simulink model "Modelo_Red_Mitigación_final"  (R2019b)
settings: Solver=VariableStepAuto  StartTime=0.0  StopTime=2.5  RelTol=1e-3
InitFcn:
  | Ts=20e-6;
undefined symbols (not defined in the file): D1, Delta, Ion, Lithium
libraries: powerlib x371, powerlib_meascontrol x286, simulink x50, simulink_extras x20, electricdrivelib x16
(part 3 of 11)

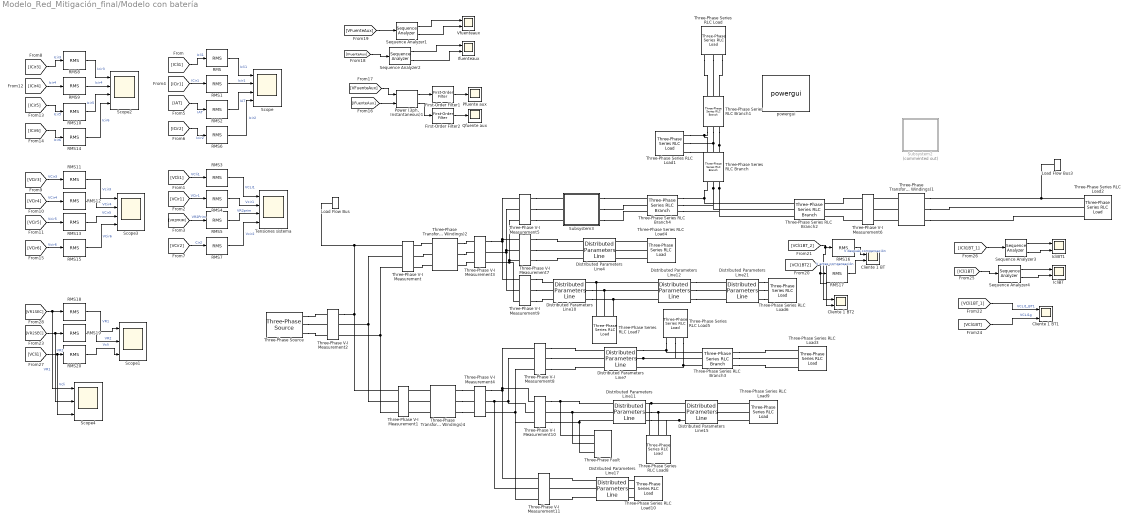
== system Modelo_Red_Mitigación_final/Modelo con batería  ==
  Cliente 1 BT : Scope  NumInputPorts=2
  Cliente 1 BT1 : Scope  NumInputPorts=3
  Cliente 1 BT2 : Scope  NumInputPorts=2
  Distributed Parameters Line10 : powerlib/Elements/Distributed Parameters Line  Phases=3  Frequency=60  Resistance=[0.213 0.639]  Inductance=[0.78e-3 2.35e-3]  Capacitance=[15e-9 15e-9]  Length=3  x1=[-2e-05 9.51822686756728e-10 32175.0070560474 -19325.063497857;-1e-05 9.56131340285843e-10 32247.6320174616 -19203.6295402535]  x2=[-2e-05 1.13231714803774e-09 31687.8811035516 -19346.7961292868;-1e-05 1.13823882988068e-09 31760.591456431 -19227.1984344754]  x3=[-2e-05 -7.26463476798207e-11 -137.471205101206 265.134927538951;-1e-05 -7.21901893651273e-11 -138.469760977224 264.614790455811]  x4=[-2e-05 7.73347694618198e-11 416.61303195894 -434.907199033177;-1e-05 7.69019064350013e-11 418.249629092397 -433.333518127755]  x5=1.78115131305569e-05  V1=ones(3,3)  V2=ones(3,3)  I1=ones(3,3)  I2=ones(3,3)  nHarmo=1  Measurements=None
      settings: SourceProductName=Simscape Electrical
  Distributed Parameters Line11 : powerlib/Elements/Distributed Parameters Line  Phases=3  Frequency=60  Resistance=[0.269 0.807]  Inductance=[0.85e-3 2.56e-3]  Capacitance=[15e-9 15e-9]  Length=18  x1=[-0.00012 -6.37664577338135e-10 31483.0427639002 -20454.4474545777;-0.00011 -6.37629545062547e-10 31559.9303096112 -20335.6141091962;-0.0001 -6.37585450659726e-10 31636.3693188544 -20216.4917497253;-9e-05 -6.37532294756353e-10 31712.3587052623 -20097.0820691573;-8e-05 -6.37470078107891e-10 31787.8973888575 -19977.3867645681;-7e-05 -6.37398801598575e-10 31862.9842960682 -19857.4075370929;-6e-05 -6.37318466241403e-10 31937.6183597431 -19737.1460919021;-5e-05 -6.37229073178117e-10 32011.7985191671 -19616.6041381771;-4e-05 -6.37130623679192e-10 32085.5237200758 -19495.7833890858;-3e-05 -6.37023119143813e-10 32158.792914671 -19374.6855617586;-2e-05 -6.36906561099856e-10 32231.6050616352 -19253.3123772635;-1e-05 -6.3678095120387e-10 32303.9591261466 -19131.6655605823]  x2=[-0.00012 -5.84352835995597e-10 29675.6367944872 -20128.6580942028;-0.00011 -5.8405713800106e-10 29751.3089897738 -20016.6408077542;-0.0001 -5.83753139261779e-10 29826.5583531049 -19904.3390405328;-9e-05 -5.83440844098248e-10 29901.3838150206 -19791.7543885953;-8e-05 -5.83120256948873e-10 29975.7843120855 -19678.8884520187;-7e-05 -5.82791382369907e-10 30049.7587869036 -19565.7428348779;-6e-05 -5.82454225035385e-10 30123.3061881342 -19452.3191452226;-5e-05 -5.8210878973706e-10 30196.4254705057 -19338.6189950544;-4e-05 -5.81755081384333e-10 30269.1155948313 -19224.6440003042;-3e-05 -5.81393105004181e-10 30341.3755280234 -19110.3957808088;-2e-05 -5.8102286574109e-10 30413.2042431086 -18995.8759602885;-1e-05 -5.80644368856979e-10 30484.6007192416 -18881.0861663232]  x3=[-0.00012 -2.40772351591986e-12 9.28421720698583 123.31084899492;-0.00011 -2.39518510900215e-12 8.81928138471592 123.344973326243;-0.0001 -2.38261266120228e-12 8.354220220936 123.37734465247;-9e-05 -2.37000635120258e-12 7.88904032519463 123.407962513534;-8e-05 -2.3573663581666e-12 7.42374830872781 123.436826474286;-7e-05 -2.34469286173662e-12 6.95835078436502 123.463936124505;-6e-05 -2.3319860420311e-12 6.49285436643523 123.489291078905;-5e-05 -2.31924607964205e-12 6.02726567067293 123.512890977134;-4e-05 -2.30647315563255e-12 5.56159131412406 123.534735483786;-3e-05 -2.29366745153411e-12 5.09583791505201 123.554824288401;-2e-05 -2.28082914934415e-12 4.63001209284352 123.573157105475;-1e-05 -2.26795843152334e-12 4.16412046791464 123.589733674456]  x4=[-0.00012 -5.10418440144233e-13 241.702417431104 -294.296225052447;-0.00011 -5.2378075498003e-13 242.810167870242 -293.382939263662;-0.0001 -5.37135625731908e-13 243.914467439433 -292.465483853906;-9e-05 -5.50482862597592e-13 245.015300444135 -291.54387186225;-8e-05 -5.63822275883302e-13 246.112651239076 -290.618116386841;-7e-05 -5.77153676006447e-13 247.206504228471 -289.688230584714;-6e-05 -5.90476873498324e-13 248.296843866248 -288.754227671603;-5e-05 -6.03791679006805e-13 249.383654656268 -287.816120921758;-4e-05 -6.17097903299031e-13 250.466921152542 -286.873923667753;-3e-05 -6.30395357264102e-13 251.546627959458 -285.927649300295;-2e-05 -6.43683851915763e-13 252.62275973199 -284.977311268038;-1e-05 -6.5696319839509e-13 253.695301175924 -284.02292307739]  x5=0.000111541920370774  V1=ones(3,3)  V2=ones(3,3)  I1=ones(3,3)  I2=ones(3,3)  nHarmo=1  Measurements=None
      settings: SourceProductName=Simscape Electrical
  Distributed Parameters Line12 : powerlib/Elements/Distributed Parameters Line  Phases=3  Frequency=60  Resistance=[0.269 0.807]  Inductance=[0.85e-3 2.56e-3]  Capacitance=[15e-9 15e-9]  Length=6  x1=[-4e-05 1.12225551603288e-09 0 0;-3e-05 1.12820660384581e-09 31614.7203957403 -19466.1188633009;-2e-05 1.1341416573456e-09 31687.8811035516 -19346.7961292868;-1e-05 1.14006059218202e-09 31760.591456431 -19227.1984344754]  x2=[-4e-05 8.82977482669238e-10 0 0;-3e-05 8.896258470369e-10 30837.5027565975 -19380.3404703214;-2e-05 8.96261567852084e-10 30910.3456112432 -19263.9483803878;-1e-05 9.0288455080651e-10 30982.7491614575 -19147.2825071068]  x3=[-4e-05 -3.70011263341918e-11 0 0;-3e-05 -3.70159507502131e-11 -40.5019848242572 176.337783353315;-2e-05 -3.70302490876394e-11 -41.1664732198487 176.183841754301;-1e-05 -3.70440211432594e-11 -41.8303765487335 176.027396192912]  x4=[-4e-05 3.94498278114461e-11 0 0;-3e-05 3.94988779511581e-11 300.866672819828 -339.753955836193;-2e-05 3.95473667243833e-11 302.145374033219 -338.617303560145;-1e-05 3.95952934419892e-11 303.419781092044 -337.475838782682]  x5=3.71806401235912e-05  V1=ones(3,3)  V2=ones(3,3)  I1=ones(3,3)  I2=ones(3,3)  nHarmo=1  Measurements=None
      settings: SourceProductName=Simscape Electrical
  Distributed Parameters Line15 : powerlib/Elements/Distributed Parameters Line  Phases=3  Frequency=60  Resistance=[0.269 0.807]  Inductance=[0.85e-3 2.56e-3]  Capacitance=[15e-9 15e-9]  Length=12  x1=[-8e-05 -5.81290096062597e-10 0 0;-7e-05 -5.80962527082388e-10 0 0;-6e-05 -5.80626701338705e-10 0 0;-5e-05 -5.80282623604376e-10 30196.4254705057 -19338.6189950544;-4e-05 -5.79930298769507e-10 30269.1155948313 -19224.6440003042;-3e-05 -5.79569731841414e-10 30341.3755280234 -19110.3957808088;-2e-05 -5.7920092794455e-10 30413.2042431086 -18995.8759602885;-1e-05 -5.78823892320436e-10 30484.6007192416 -18881.0861663232]  x2=[-8e-05 -5.1837948200219e-10 0 0;-7e-05 -5.17954517458826e-10 0 0;-6e-05 -5.17522191635274e-10 0 0;-5e-05 -5.17082510675841e-10 29816.1536069767 -19273.9878791668;-4e-05 -5.16635480829367e-10 29888.6027805653 -19161.4469314478;-3e-05 -5.16181108449134e-10 29960.6271709498 -19048.633657154;-2e-05 -5.15719399992781e-10 30032.2257545041 -18935.5496596116;-1e-05 -5.15250362022206e-10 30103.3975136541 -18822.1965459946]  x3=[-8e-05 6.30193856587518e-13 0 0;-7e-05 6.47027122188518e-13 0 0;-6e-05 6.63851192101914e-13 0 0;-5e-05 6.80665827220432e-13 86.3403246372238 -15.5892894445521;-4e-05 6.97470788570887e-13 86.3984811910831 -15.2636840808927;-3e-05 7.14265837317582e-13 86.4554098312811 -14.9378617864961;-2e-05 7.31050734765698e-13 86.511109748736 -14.6118271920186;-1e-05 7.47825242364687e-13 86.5655801518285 -14.2855849311333]  x4=[-8e-05 -2.76869898482782e-12 0 0;-7e-05 -2.78266132861739e-12 0 0;-6e-05 -2.79658412463005e-12 0 0;-5e-05 -2.81046717499204e-12 161.912076262647 -146.998141908733;-4e-05 -2.82431028239449e-12 162.465094324739 -146.38670462291;-3e-05 -2.8381132500962e-12 163.015803398223 -145.773186857987;-2e-05 -2.85187588192645e-12 163.564195656305 -145.157597333408;-1e-05 -2.86559798228777e-12 164.110263305116 -144.539944798065]  x5=7.43612802471824e-05  V1=ones(3,3)  V2=ones(3,3)  I1=ones(3,3)  I2=ones(3,3)  nHarmo=1  Measurements=None
      settings: SourceProductName=Simscape Electrical
  Distributed Parameters Line17 : powerlib/Elements/Distributed Parameters Line  Phases=3  Frequency=60  Resistance=[0.213 0.639]  Inductance=[0.78e-3 2.35e-3]  Capacitance=[15e-9 15e-9]  Length=18  x1=[-0.00011 -6.37629545062547e-10 31559.9303096112 -20335.6141091962;-0.0001 -6.37585450659726e-10 31636.3693188544 -20216.4917497253;-9e-05 -6.37532294756353e-10 31712.3587052623 -20097.0820691573;-8e-05 -6.37470078107891e-10 31787.8973888575 -19977.3867645681;-7e-05 -6.37398801598575e-10 31862.9842960682 -19857.4075370929;-6e-05 -6.37318466241403e-10 31937.6183597431 -19737.1460919021;-5e-05 -6.37229073178117e-10 32011.7985191671 -19616.6041381771;-4e-05 -6.37130623679192e-10 32085.5237200758 -19495.7833890858;-3e-05 -6.37023119143813e-10 32158.792914671 -19374.6855617586;-2e-05 -6.36906561099856e-10 32231.6050616352 -19253.3123772635;-1e-05 -6.3678095120387e-10 32303.9591261466 -19131.6655605823]  x2=[-0.00011 -5.81093394391643e-10 30839.7793585654 -20381.2716559516;-0.0001 -5.80562463791867e-10 30916.3956097666 -20264.8638707272;-9e-05 -5.80023282114402e-10 30992.5724705526 -20148.1680769308;-8e-05 -5.79475857022214e-10 31068.3088582815 -20031.1859330679;-7e-05 -5.78920196295424e-10 31143.6036965717 -19913.9191017138;-6e-05 -5.78356307831202e-10 31218.4559153168 -19796.3692494898;-5e-05 -5.77784199643652e-10 31292.8644507012 -19678.5380470393;-4e-05 -5.77203879863696e-10 31366.8282452148 -19560.4271690046;-3e-05 -5.76615356738963e-10 31440.3462476684 -19442.0382940027;-2e-05 -5.7601863863367e-10 31513.4174132084 -19323.3731046016;-1e-05 -5.75413734028501e-10 31586.0407033319 -19204.4332872963]  x3=[-0.00011 -5.33423696024894e-12 65.9317893508074 -5.21472769212498;-0.0001 -5.30896708029375e-12 65.9509798461571 -4.96613423439622;-9e-05 -5.28362174816493e-12 65.9692330321003 -4.71747019690742;-8e-05 -5.25820132407573e-12 65.9865486492189 -4.46873911372498;-7e-05 -5.23270616930667e-12 66.0029264514196 -4.21994451986815;-6e-05 -5.20713664620032e-12 66.0183662059376 -3.97108995125883;-5e-05 -5.1814931181562e-12 66.0328676933398 -3.72217894467127;-4e-05 -5.15577594962561e-12 66.046430707528 -3.47321503768184;-3e-05 -5.12998550610644e-12 66.0590550557418 -3.22420176861875;-2e-05 -5.10412215413798e-12 66.0707405585611 -2.97514267651174;-1e-05 -5.0781862612957e-12 66.0814870499091 -2.72604130104181]  x4=[-0.00011 2.08995199063691e-12 202.227351702482 -174.253957712764;-0.0001 2.06944266433478e-12 202.882835041371 -173.490342096433;-9e-05 2.04890392667166e-12 203.535434966092 -172.724260798319;-8e-05 2.02833606954849e-12 204.185142201756 -171.955724706133;-7e-05 2.00773938528004e-12 204.831947514583 -171.184744742474;-6e-05 1.98711416659078e-12 205.47584171204 -170.411331864673;-5e-05 1.96646070661072e-12 206.116815642964 -169.635497064641;-4e-05 1.94577929887126e-12 206.754860197698 -168.857251368706;-3e-05 1.92507023730096e-12 207.389966308214 -168.076605837463;-2e-05 1.90433381622144e-12 208.022124948251 -167.293571565612;-1e-05 1.88357033034313e-12 208.651327133435 -166.508159681805]  x5=0.000106869078783341  V1=ones(3,3)  V2=ones(3,3)  I1=ones(3,3)  I2=ones(3,3)  nHarmo=1  Measurements=None
      settings: SourceProductName=Simscape Electrical
  Distributed Parameters Line21 : powerlib/Elements/Distributed Parameters Line  Phases=3  Frequency=60  Resistance=[0.269 0.807]  Inductance=[0.85e-3 2.56e-3]  Capacitance=[15e-9 15e-9]  Length=3  x1=[-2e-05 8.96265853704287e-10 30910.3456112432 -19263.9483803878;-1e-05 9.02886693747839e-10 30982.7491614575 -19147.2825071068]  x2=[-2e-05 8.82848388597059e-10 30521.2143172031 -19221.4149453175;-1e-05 8.88901904202634e-10 30593.4602857332 -19106.2163612263]  x3=[-2e-05 3.05576494227813e-11 -43.7280619985849 177.821448028189;-1e-05 3.04685047093702e-11 -44.3981207401299 177.655333890483]  x4=[-2e-05 -2.43827173429009e-11 300.811121285802 -339.602032284589;-1e-05 -2.42495845607924e-11 302.089250157008 -338.465590511979]  x5=1.85903200617956e-05  V1=ones(3,3)  V2=ones(3,3)  I1=ones(3,3)  I2=ones(3,3)  nHarmo=1  Measurements=None
      settings: SourceProductName=Simscape Electrical
  Distributed Parameters Line4 : powerlib/Elements/Distributed Parameters Line  Phases=3  Frequency=60  Resistance=[0.213 0.639]  Inductance=[0.78e-3 2.35e-3]  Capacitance=[15e-9 15e-9]  Length=9  x1=[-6e-05 9.27062321547884e-10 31879.9448487023 -19808.0356092313;-5e-05 9.31443643683125e-10 31954.3926645116 -19687.7105752571;-4e-05 9.35811727942434e-10 32028.3863376699 -19567.1057353368;-3e-05 9.40166512245665e-10 32101.9248165634 -19446.2228035321;-2e-05 9.44507934701694e-10 32175.0070560474 -19325.063497857;-1e-05 9.48835933609296e-10 32247.6320174616 -19203.6295402535]  x2=[-6e-05 9.30715846640024e-10 31220.754132217 -19854.1863402283;-5e-05 9.36913847546258e-10 31295.3806160507 -19736.3460628703;-4e-05 9.43098532832856e-10 31369.5623232534 -19618.2252883483;-3e-05 9.49269814601747e-10 31443.2981995388 -19499.8256954198;-2e-05 9.5542760514536e-10 31516.5871969568 -19381.1489668053;-1e-05 9.61571816947859e-10 31589.4282739087 -19262.1967891637]  x3=[-6e-05 -3.66911385239073e-11 9.19435123998005 67.3100361697751;-5e-05 -3.65713742858999e-11 8.94053364683108 67.3442196629408;-4e-05 -3.64510902877129e-11 8.68658898890908 67.3774460456783;-3e-05 -3.63302882388482e-11 8.43252087532973 67.4097148457672;-2e-05 -3.62089698561704e-11 8.17833291696331 67.4410256045963;-1e-05 -3.60871368638822e-11 7.92402872638336 67.4713778771705]  x4=[-6e-05 4.05346197813055e-11 264.776860672235 -241.746580654789;-5e-05 4.04416044214767e-11 265.686340119028 -240.74667989379;-4e-05 4.03480142969314e-11 266.59204357483 -239.743357589577;-3e-05 4.02538507377923e-11 267.49395816759 -238.736628001579;-2e-05 4.01591150823322e-11 268.392071079105 -237.726505437652;-1e-05 4.00638086769543e-11 269.286369545202 -236.713004253875]  x5=5.34345393916706e-05  V1=ones(3,3)  V2=ones(3,3)  I1=ones(3,3)  I2=ones(3,3)  nHarmo=1  Measurements=None
      settings: SourceProductName=Simscape Electrical
  Distributed Parameters Line7 : powerlib/Elements/Distributed Parameters Line  Phases=3  Frequency=60  Resistance=[0.213 0.639]  Inductance=[0.78e-3 2.35e-3]  Capacitance=[15e-9 15e-9]  Length=4.4  x1=[-3e-05 -6.37023119143813e-10 0 0;-2e-05 -6.36906561099856e-10 32231.6050616352 -19253.3123772635;-1e-05 -6.3678095120387e-10 32303.9591261466 -19131.6655605823]  x2=[-3e-05 -6.20206594908238e-10 0 0;-2e-05 -6.19631999252479e-10 31928.0322823366 -19306.2030459998;-1e-05 -6.19048597254452e-10 32000.58789672 -19185.700293177]  x3=[-3e-05 -2.2707610684769e-11 0 0;-2e-05 -2.26378782855031e-11 2.67417656215666 49.6193899931641;-1e-05 -2.25678241518777e-11 2.48709730897001 49.6291187767325]  x4=[-3e-05 1.89896750235836e-11 0 0;-2e-05 1.89284208409242e-11 277.339936666534 -218.99027498491;-1e-05 1.88668976435065e-11 278.163537790718 -217.943174364135]  x5=2.61235525914834e-05  V1=ones(3,3)  V2=ones(3,3)  I1=ones(3,3)  I2=ones(3,3)  nHarmo=1  Measurements=None
      settings: SourceProductName=Simscape Electrical
  First-Order Filter1 : powerlib_meascontrol/Filters/First-Order Filter  FilterType=Lowpass  Tc=10e-3  Ts=0  Initialize=on  Vac_Init=[0, 0, 60]  Vdc_Init=0  PlotResponse=off  FreqRange="[0,  200,  1]"
      settings: SourceProductName=Simscape Electrical
  First-Order Filter2 : powerlib_meascontrol/Filters/First-Order Filter  FilterType=Lowpass  Tc=10e-3  Ts=0  Initialize=on  Vac_Init=[0, 0, 60]  Vdc_Init=0  PlotResponse=off  FreqRange="[0,  200,  1]"
      settings: SourceProductName=Simscape Electrical
  IcliBT : Scope  NumInputPorts=2
  IcliBT1 : Scope  NumInputPorts=2
  Ifuenteaux : Scope  NumInputPorts=2
  Load Flow Bus : powerlib/Measurements/Load Flow Bus  LConnTagsString=a  Phases=single  Connectors=on one side  ID=BUS_1  Vbase=115e3  Vref=1.05  Vangle=0  VLF=1  VLFb=1  VLFc=1  angleLF=0  angleLFb=0  angleLFc=0
      settings: SourceProductName=Simscape Electrical
  Load Flow Bus3 : powerlib/Measurements/Load Flow Bus  LConnTagsString=a  Phases=single  Connectors=on one side  ID=BUS_4  Vbase=440  Vref=1  Vangle=0  VLF=0.9785  VLFb=1  VLFc=1  angleLF=28.33  angleLFb=0  angleLFc=0
      settings: SourceProductName=Simscape Electrical
  "Pfuente aux " : Scope
  "Power (3ph, Instantaneous)1" : powerlib_meascontrol/Measurements/Power (3ph, Instantaneous)
      settings: SourceProductName=Simscape Electrical
  Qfuente aux : Scope
  RMS{,1..20} (21 alike) : powerlib_meascontrol/Measurements/RMS  TrueRMS=on  Freq=60  RMSInit=120  Ts=0
      settings: SourceProductName=Simscape Electrical
  Scope : Scope  NumInputPorts=4
  Scope1 : Scope  NumInputPorts=3
  Scope2 : Scope  NumInputPorts=4
  Scope3 : Scope  NumInputPorts=4
  Scope4 : Scope  NumInputPorts=3
  Sequence Analyzer{1..4} (4 alike) : powerlib_meascontrol/Measurements/Sequence Analyzer  Freq=60  n=1  seq=Positive Negative Zero  InInit=[1, 0]  Ts=0
      settings: SourceProductName=Simscape Electrical  SourceProductBaseCode=PS
  Subsystem2 : Subsystem  Commented=on
  Subsystem3 : Subsystem
  Tensiones sistema : Scope  NumInputPorts=4
  Three-Phase Series RLC Branch : powerlib/Elements/Three-Phase Series RLC Branch  LConnTagsString=A|B|C  RConnTagsString=A|B|C  BranchType=RL  Resistance=0.213  Inductance=0.78e-3  Capacitance=1e-6  Measurements=None
      settings: SourceProductName=Simscape Electrical
  Three-Phase Series RLC Branch1 : powerlib/Elements/Three-Phase Series RLC Branch  LConnTagsString=A|B|C  RConnTagsString=A|B|C  BranchType=RL  Resistance=0.213  Inductance=0.78e-3  Capacitance=1e-6  Measurements=None
      settings: SourceProductName=Simscape Electrical
  Three-Phase Series RLC Branch2 : powerlib/Elements/Three-Phase Series RLC Branch  LConnTagsString=A|B|C  RConnTagsString=A|B|C  BranchType=RL  Resistance=0.213*1.7  Inductance=0.78e-3*1.7  Capacitance=1e-6  Measurements=None
      settings: SourceProductName=Simscape Electrical
  Three-Phase Series RLC Branch3 : powerlib/Elements/Three-Phase Series RLC Branch  LConnTagsString=A|B|C  RConnTagsString=A|B|C  BranchType=RL  Resistance=0.213*2.2  Inductance=0.78e-3*2.2  Capacitance=1e-6  Measurements=None
      settings: SourceProductName=Simscape Electrical
  Three-Phase Series RLC Branch4 : powerlib/Elements/Three-Phase Series RLC Branch  LConnTagsString=A|B|C  RConnTagsString=A|B|C  BranchType=RL  Resistance=0.213*7  Inductance=0.78e-3*7  Capacitance=1e-6  Measurements=None
      settings: SourceProductName=Simscape Electrical
  Three-Phase Series RLC Load : powerlib/Elements/Three-Phase Series RLC Load  LConnTagsString=A|B|C  Configuration=Y (grounded)  NominalVoltage=34.5e3  Vabc=[1e3 1e3 1e3]  Vabcp=[1e3 1e3 1e3]  NominalFrequency=60  UnbalancedPower=off  ActivePower=0.5e6  InductivePower=0.1e6  CapacitivePower=0  Pabc=[10e3 9e3 11e3]  QLabc=[100 90 110]  QCabc=[100 90 110]  Pabcp=[10e3 9e3 11e3]  QLabcp=[100 90 110]  QCabcp=[100 90 110]  Measurements=None  LoadType=constant Z
      settings: SourceProductName=Simscape Electrical
  Three-Phase Series RLC Load1 : powerlib/Elements/Three-Phase Series RLC Load  LConnTagsString=A|B|C  Configuration=Y (grounded)  NominalVoltage=34.5e3  Vabc=[1e3 1e3 1e3]  Vabcp=[1e3 1e3 1e3]  NominalFrequency=60  UnbalancedPower=off  ActivePower=2.5e6  InductivePower=1e6  CapacitivePower=0  Pabc=[10e3 9e3 11e3]  QLabc=[100 90 110]  QCabc=[100 90 110]  Pabcp=[10e3 9e3 11e3]  QLabcp=[100 90 110]  QCabcp=[100 90 110]  Measurements=None  LoadType=constant Z
      settings: SourceProductName=Simscape Electrical
  Three-Phase Series RLC Load10 : powerlib/Elements/Three-Phase Series RLC Load  LConnTagsString=A|B|C  Configuration=Y (grounded)  NominalVoltage=34.5e3  Vabc=[1e3 1e3 1e3]  Vabcp=[1e3 1e3 1e3]  NominalFrequency=60  UnbalancedPower=off  ActivePower=3.4e6  InductivePower=1.1e6  CapacitivePower=0  Pabc=[10e3 9e3 11e3]  QLabc=[100 90 110]  QCabc=[100 90 110]  Pabcp=[10e3 9e3 11e3]  QLabcp=[100 90 110]  QCabcp=[100 90 110]  Measurements=None  LoadType=constant Z
      settings: SourceProductName=Simscape Electrical
  Three-Phase Series RLC Load2 : powerlib/Elements/Three-Phase Series RLC Load  LConnTagsString=A|B|C  Configuration=Y (grounded)  NominalVoltage=440  Vabc=[1e3 1e3 1e3]  Vabcp=[1e3 1e3 1e3]  NominalFrequency=60  UnbalancedPower=off  ActivePower=6.5e6  InductivePower=3e6  CapacitivePower=0  Pabc=[10e3 9e3 11e3]  QLabc=[100 90 110]  QCabc=[100 90 110]  Pabcp=[10e3 9e3 11e3]  QLabcp=[100 90 110]  QCabcp=[100 90 110]  Measurements=None  LoadType=constant Z
      settings: SourceProductName=Simscape Electrical
  Three-Phase Series RLC Load3 : powerlib/Elements/Three-Phase Series RLC Load  LConnTagsString=A|B|C  Configuration=Y (grounded)  NominalVoltage=34.5e3  Vabc=[1e3 1e3 1e3]  Vabcp=[1e3 1e3 1e3]  NominalFrequency=60  UnbalancedPower=off  ActivePower=3e6  InductivePower=0.7e6  CapacitivePower=0  Pabc=[10e3 9e3 11e3]  QLabc=[100 90 110]  QCabc=[100 90 110]  Pabcp=[10e3 9e3 11e3]  QLabcp=[100 90 110]  QCabcp=[100 90 110]  Measurements=None  LoadType=constant Z
      settings: SourceProductName=Simscape Electrical
  Three-Phase Series RLC Load4 : powerlib/Elements/Three-Phase Series RLC Load  LConnTagsString=A|B|C  Configuration=Y (grounded)  NominalVoltage=34.5e3  Vabc=[1e3 1e3 1e3]  Vabcp=[1e3 1e3 1e3]  NominalFrequency=60  UnbalancedPower=off  ActivePower=6.2e6  InductivePower=2e6  CapacitivePower=0  Pabc=[10e3 9e3 11e3]  QLabc=[100 90 110]  QCabc=[100 90 110]  Pabcp=[10e3 9e3 11e3]  QLabcp=[100 90 110]  QCabcp=[100 90 110]  Measurements=None  LoadType=constant Z
      settings: SourceProductName=Simscape Electrical
  Three-Phase Series RLC Load5 : powerlib/Elements/Three-Phase Series RLC Load  LConnTagsString=A|B|C  Configuration=Y (grounded)  NominalVoltage=34.5e3  Vabc=[1e3 1e3 1e3]  Vabcp=[1e3 1e3 1e3]  NominalFrequency=60  UnbalancedPower=off  ActivePower=3e6  InductivePower=0.7e6  CapacitivePower=0  Pabc=[10e3 9e3 11e3]  QLabc=[100 90 110]  QCabc=[100 90 110]  Pabcp=[10e3 9e3 11e3]  QLabcp=[100 90 110]  QCabcp=[100 90 110]  Measurements=None  LoadType=constant Z
      settings: SourceProductName=Simscape Electrical
  Three-Phase Series RLC Load6 : powerlib/Elements/Three-Phase Series RLC Load  LConnTagsString=A|B|C  Configuration=Y (grounded)  NominalVoltage=34.5e3  Vabc=[1e3 1e3 1e3]  Vabcp=[1e3 1e3 1e3]  NominalFrequency=60  UnbalancedPower=off  ActivePower=9.4e6  InductivePower=4.2e6  CapacitivePower=0  Pabc=[10e3 9e3 11e3]  QLabc=[100 90 110]  QCabc=[100 90 110]  Pabcp=[10e3 9e3 11e3]  QLabcp=[100 90 110]  QCabcp=[100 90 110]  Measurements=None  LoadType=constant Z
      settings: SourceProductName=Simscape Electrical
  Three-Phase Series RLC Load7 : powerlib/Elements/Three-Phase Series RLC Load  LConnTagsString=A|B|C  Configuration=Y (grounded)  NominalVoltage=34.5e3  Vabc=[1e3 1e3 1e3]  Vabcp=[1e3 1e3 1e3]  NominalFrequency=60  UnbalancedPower=off  ActivePower=4.4e6  InductivePower=0.8e6  CapacitivePower=0  Pabc=[10e3 9e3 11e3]  QLabc=[100 90 110]  QCabc=[100 90 110]  Pabcp=[10e3 9e3 11e3]  QLabcp=[100 90 110]  QCabcp=[100 90 110]  Measurements=None  LoadType=constant Z
      settings: SourceProductName=Simscape Electrical
  Three-Phase Series RLC Load8 : powerlib/Elements/Three-Phase Series RLC Load  LConnTagsString=A|B|C  Configuration=Y (grounded)  NominalVoltage=34.5e3  Vabc=[1e3 1e3 1e3]  Vabcp=[1e3 1e3 1e3]  NominalFrequency=60  UnbalancedPower=off  ActivePower=5e6  InductivePower=2.5e6  CapacitivePower=0  Pabc=[10e3 9e3 11e3]  QLabc=[100 90 110]  QCabc=[100 90 110]  Pabcp=[10e3 9e3 11e3]  QLabcp=[100 90 110]  QCabcp=[100 90 110]  Measurements=None  LoadType=constant Z
      settings: SourceProductName=Simscape Electrical
  Three-Phase Series RLC Load9 : powerlib/Elements/Three-Phase Series RLC Load  LConnTagsString=A|B|C  Configuration=Y (grounded)  NominalVoltage=34.5e3  Vabc=[1e3 1e3 1e3]  Vabcp=[1e3 1e3 1e3]  NominalFrequency=60  UnbalancedPower=off  ActivePower=2.3e6  InductivePower=1.2e6  CapacitivePower=0  Pabc=[10e3 9e3 11e3]  QLabc=[100 90 110]  QCabc=[100 90 110]  Pabcp=[10e3 9e3 11e3]  QLabcp=[100 90 110]  QCabcp=[100 90 110]  Measurements=None  LoadType=constant Z
      settings: SourceProductName=Simscape Electrical
  Three-Phase V-I Measurement : powerlib/Measurements/Three-Phase V-I Measurement  VoltageMeasurement=phase-to-ground  SetLabelV=on  LabelV=VR2PRIM  Vpu=off  VpuLL=off  CurrentMeasurement=yes  SetLabelI=on  LabelI=IR2PRIM  Ipu=off  Pbase=100e6  Vbase=500e3  OutputType=Complex  PhasorSimulation=off  PSBequivalent=0
      settings: SourceProductName=Simscape Electrical
  Three-Phase V-I Measurement1 : powerlib/Measurements/Three-Phase V-I Measurement  VoltageMeasurement=phase-to-ground  SetLabelV=on  LabelV=VR1PRIM  Vpu=off  VpuLL=off  CurrentMeasurement=yes  SetLabelI=on  LabelI=IR1PRIM  Ipu=off  Pbase=100e6  Vbase=500e3  OutputType=Complex  PhasorSimulation=off  PSBequivalent=0
      settings: SourceProductName=Simscape Electrical
  Three-Phase V-I Measurement10 : powerlib/Measurements/Three-Phase V-I Measurement  VoltageMeasurement=phase-to-ground  SetLabelV=on  LabelV=VCir5  Vpu=off  VpuLL=off  CurrentMeasurement=yes  SetLabelI=on  LabelI=ICir5  Ipu=off  Pbase=100e6  Vbase=500e3  OutputType=Complex  PhasorSimulation=off  PSBequivalent=0
      settings: SourceProductName=Simscape Electrical
  Three-Phase V-I Measurement11 : powerlib/Measurements/Three-Phase V-I Measurement  VoltageMeasurement=phase-to-ground  SetLabelV=on  LabelV=VCir6  Vpu=off  VpuLL=off  CurrentMeasurement=yes  SetLabelI=on  LabelI=ICir6  Ipu=off  Pbase=100e6  Vbase=500e3  OutputType=Complex  PhasorSimulation=off  PSBequivalent=0
      settings: SourceProductName=Simscape Electrical
  Three-Phase V-I Measurement2 : powerlib/Measurements/Three-Phase V-I Measurement  VoltageMeasurement=phase-to-ground  SetLabelV=on  LabelV=VAT  Vpu=off  VpuLL=off  CurrentMeasurement=yes  SetLabelI=on  LabelI=IAT  Ipu=off  Pbase=100e6  Vbase=500e3  OutputType=Complex  PhasorSimulation=off  PSBequivalent=0
      settings: SourceProductName=Simscape Electrical
  Three-Phase V-I Measurement3 : powerlib/Measurements/Three-Phase V-I Measurement  VoltageMeasurement=phase-to-ground  SetLabelV=on  LabelV=VR2SEC  Vpu=off  VpuLL=off  CurrentMeasurement=yes  SetLabelI=on  LabelI=IR2SEC  Ipu=off  Pbase=100e6  Vbase=500e3  OutputType=Complex  PhasorSimulation=off  PSBequivalent=0
      settings: SourceProductName=Simscape Electrical
  Three-Phase V-I Measurement4 : powerlib/Measurements/Three-Phase V-I Measurement  VoltageMeasurement=phase-to-ground  SetLabelV=on  LabelV=VR1SEC  Vpu=off  VpuLL=off  CurrentMeasurement=yes  SetLabelI=on  LabelI=IR1SEC  Ipu=off  Pbase=100e6  Vbase=500e3  OutputType=Complex  PhasorSimulation=off  PSBequivalent=0
      settings: SourceProductName=Simscape Electrical
  Three-Phase V-I Measurement5 : powerlib/Measurements/Three-Phase V-I Measurement  VoltageMeasurement=phase-to-ground  SetLabelV=on  LabelV=VCir1  Vpu=off  VpuLL=off  CurrentMeasurement=yes  SetLabelI=on  LabelI=ICir1  Ipu=off  Pbase=100e6  Vbase=500e3  OutputType=Complex  PhasorSimulation=off  PSBequivalent=0
      settings: SourceProductName=Simscape Electrical
  Three-Phase V-I Measurement6 : powerlib/Measurements/Three-Phase V-I Measurement  VoltageMeasurement=phase-to-ground  SetLabelV=on  LabelV=VCli1  Vpu=off  VpuLL=off  CurrentMeasurement=yes  SetLabelI=on  LabelI=ICli1  Ipu=off  Pbase=100e6  Vbase=500e3  OutputType=Complex  PhasorSimulation=off  PSBequivalent=0
      settings: SourceProductName=Simscape Electrical
  Three-Phase V-I Measurement7 : powerlib/Measurements/Three-Phase V-I Measurement  VoltageMeasurement=phase-to-ground  SetLabelV=on  LabelV=VCir2  Vpu=off  VpuLL=off  CurrentMeasurement=yes  SetLabelI=on  LabelI=ICir2  Ipu=off  Pbase=100e6  Vbase=500e3  OutputType=Complex  PhasorSimulation=off  PSBequivalent=0
      settings: SourceProductName=Simscape Electrical
  Three-Phase V-I Measurement8 : powerlib/Measurements/Three-Phase V-I Measurement  VoltageMeasurement=phase-to-ground  SetLabelV=on  LabelV=VCir4  Vpu=off  VpuLL=off  CurrentMeasurement=yes  SetLabelI=on  LabelI=ICir4  Ipu=off  Pbase=100e6  Vbase=500e3  OutputType=Complex  PhasorSimulation=off  PSBequivalent=0
      settings: SourceProductName=Simscape Electrical
  Three-Phase V-I Measurement9 : powerlib/Measurements/Three-Phase V-I Measurement  VoltageMeasurement=phase-to-ground  SetLabelV=on  LabelV=VCir3  Vpu=off  VpuLL=off  CurrentMeasurement=yes  SetLabelI=on  LabelI=ICir3  Ipu=off  Pbase=100e6  Vbase=500e3  OutputType=Complex  PhasorSimulation=off  PSBequivalent=0
      settings: SourceProductName=Simscape Electrical
  Three-Phase Fault : powerlib/Elements/Three-Phase Fault  InitialStates=0  FaultA=on  FaultB=on  FaultC=on  GroundFault=off  SwitchTimes=[0.2,0.4]  External=off  SwitchStatus=NaN  FaultResistance=0.3  GroundResistance=0.01  SnubberResistance=1e6  SnubberCapacitance=inf  Measurements=None
      settings: SourceProductName=Simscape Electrical
  Three-Phase Source : powerlib/Electrical Sources/Three-Phase Source  InternalConnection=Yg  VoltagePhases=off  Voltage=(115000)*1.39942  PhaseAngle=16.7311  Voltage_phases=[25e3 25e3 25e3]/sqrt(3)  PhaseAngles_phases=[0 -120 +120]  Frequency=60  NonIdealSource=on  SpecifyImpedance=on  Resistance=0.8929  Inductance=16.58e-3  ShortCircuitLevel=100e6  BaseVoltage=115e3  XRratio=5.946  BusType=swing  Pref=10e3  Qref=0  Prefabc=[10e3, 10e3, 10e3]  Qrefabc=[0, 0, 0]  Qmin=-inf  Qmax=inf
      settings: SourceProductName=Simscape Electrical
  Three-Phase Transformer Inductance Matrix Type (Two Windings)1 : powerlib/Elements/Three-Phase Transformer Inductance Matrix Type (Two Windings)  CoreType=Three-limb or five-limb core  Winding1Connection=Yg  Winding2Connection=Yg  AutoTransformer=off  Measurements=None  NominalPower=[10e6, 60]  VLLnom=[34.5e3, 440]  WindingResistances=[0.01, 0.01]  NoLoadIexcPos=2  NoLoadPlossPos=1000  ShortCircuitReactancePos=0.06  ShortCircuitReactancePosAuto=0.06  NoLoadIexcZero=100  NoLoadPlossZero=500000  ShortCircuitReactanceZero=0.03  ShortCircuitReactanceZeroAuto=0.03
      settings: SourceProductName=Simscape Electrical  SourceProductBaseCode=PS
  Three-Phase Transformer Inductance Matrix Type (Two Windings)2 : powerlib/Elements/Three-Phase Transformer Inductance Matrix Type (Two Windings)  CoreType=Three single-phase cores  Winding1Connection=Delta (D1)  Winding2Connection=Y  AutoTransformer=off  Measurements=None  NominalPower=[40e6, 60]  VLLnom=[115e3, 34.5e3]  WindingResistances=[0.006, 0.006]  NoLoadIexcPos=2  NoLoadPlossPos=16600  ShortCircuitReactancePos=0.1056  ShortCircuitReactancePosAuto=0.06  NoLoadIexcZero=100  NoLoadPlossZero=500000  ShortCircuitReactanceZero=0.1056  ShortCircuitReactanceZeroAuto=0.03
      settings: SourceProductName=Simscape Electrical  SourceProductBaseCode=PS
  Three-Phase Transformer Inductance Matrix Type (Two Windings)4 : powerlib/Elements/Three-Phase Transformer Inductance Matrix Type (Two Windings)  CoreType=Three single-phase cores  Winding1Connection=Delta (D1)  Winding2Connection=Y  AutoTransformer=off  Measurements=None  NominalPower=[30e6, 60]  VLLnom=[115e3, 34.5e3]  WindingResistances=[0.006, 0.006]  NoLoadIexcPos=2  NoLoadPlossPos=14300  ShortCircuitReactancePos=0.0912  ShortCircuitReactancePosAuto=0.06  NoLoadIexcZero=100  NoLoadPlossZero=500000  ShortCircuitReactanceZero=0.0912  ShortCircuitReactanceZeroAuto=0.03
      settings: SourceProductName=Simscape Electrical  SourceProductBaseCode=PS
  Vfuenteaux : Scope  NumInputPorts=2
  powergui : powerlib/powergui  Priority=1  SimulationMode=Discrete  SampleTime=10e-6  frequency=60  Iterations=50  frequencyindice=0  Pbase=100e6  ErrMax=0.0001  UnitsV=kV  UnitsW=MW  buscounter=0  FunctionMessages=off  echomessages=off  EnableUseOfTLC=off  CurrentSourceSwitches=off  DisableSnubberDevices=off  DisableRonSwitches=off  DisableVfSwitches=off  DisplayEquations=off  AutomaticDiscreteSolvers=off  SolverType=Tustin/Backward Euler (TBE)  Interpol=off  ExternalGateDelay=off  methode=off  Ts=100  x0status=blocks  SPID=on  SwTol=0  HookPort=off  NonlinearTolerance=1e-4  nMaxIteration=100  ContinueOnMaxIteration=off  RestoreLinks=warning  ResistiveCurrentMeasurement=off  Frange=[0:2:500]  Ylog=off  Xlog=on  ShowGrid=off  save=off  variable=ZData  structure=0  ZoomFFT=off  StartTime=0.0  cycles=1  DisplayStyle=1  fundamental=60  FreqAxis=off  MaxFrequency=1000  frequencyindicesteady=1  RmsSteady=1  display=off
      settings: SourceProductName=Simscape Electrical
  wires:
  RMS1/1 -> Scope/2  "Icir1"
  Sequence Analyzer4/2 -> IcliBT/2
  RMS5/1 -> Tensiones sistema/3  "VR2prim"
  [VCli1] -> RMS3/1  "VCli1"
  "Power (3ph, Instantaneous)1"/2 -> First-Order Filter2/1
  RMS13/1 -> Scope3/3  "VCir5"
  [ICir5] -> RMS10/1  "Icir5"
  Sequence Analyzer1/2 -> Vfuenteaux/2
  [ICir2] -> RMS6/1  "Icir2"
  RMS7/1 -> Tensiones sistema/4  "Vcir2"
  Sequence Analyzer3/1 -> IcliBT1/1
  Sequence Analyzer4/1 -> IcliBT/1
  RMS9/1 -> Scope2/2  "Icir4"
  [VCir3] -> RMS11/1  "VCir3"
  [VFuenteAux] -> Sequence Analyzer1/1
  [VCir5] -> RMS13/1  "Vcir5"
  [VCli1BT2] -> Cliente 1 BT2/2, RMS17/1
  [ICir1] -> RMS1/1  "ICir1"
  [VCir6] -> RMS15/1  "Vcir6"
  [ICli1BT] -> Sequence Analyzer4/1
  First-Order Filter1/1 -> "Pfuente aux "/1
  RMS3/1 -> Tensiones sistema/1  "VCLI1"
  [VCli1BT] -> Cliente 1 BT1/3  "VCLI1g"
  Sequence Analyzer3/2 -> IcliBT1/2
  Sequence Analyzer2/1 -> Ifuenteaux/1
  [VCli1BT_1] -> Cliente 1 BT1/1  "VCLI1_BT1"
  RMS17/1 -> Cliente 1 BT/2  "V antes compensación"
  RMS16/1 -> Cliente 1 BT/1  "V después compensación"
  [VCir2] -> RMS7/1  "Cir2"
  [ICli1BT_1] -> Sequence Analyzer3/1
  RMS14/1 -> Scope2/4  "Icir6"
  First-Order Filter2/1 -> Qfuente aux/1
  RMS6/1 -> Scope/4  "Icir2"
  RMS/1 -> Scope/1  "Icli1"
  [ICli1] -> RMS/1  "Icli1"
  [VCir1] -> RMS4/1  "VCir1"
  RMS4/1 -> Tensiones sistema/2  "Vcir1"
  [VR2PRIM] -> RMS5/1  "VR2Prim"
  [ICir6] -> RMS14/1  "Icir6"
  [IAT] -> RMS2/1  "IAT"
  RMS2/1 -> Scope/3  "IAT"
  RMS15/1 -> Scope3/4  "VCir6"
  [ICir3] -> RMS8/1  "Icir3"
  [VCir4] -> RMS12/1  "VCir4"
  [ICir4] -> RMS9/1  "Icir4"
  [VFuenteAux] -> "Power (3ph, Instantaneous)1"/1
  RMS12/1 -> Scope3/2  "VCir4"
  RMS10/1 -> Scope2/3  "Icir5"
  [IFuenteAux] -> "Power (3ph, Instantaneous)1"/2
  RMS11/1 -> Scope3/1  "Vcir3"
  "Power (3ph, Instantaneous)1"/1 -> First-Order Filter1/1
  RMS8/1 -> Scope2/1  "Icir3"
  [IFuenteAux] -> Sequence Analyzer2/1
  Sequence Analyzer2/2 -> Ifuenteaux/2
  Sequence Analyzer1/1 -> Vfuenteaux/1
  [VCli1BT_2] -> Cliente 1 BT2/1, RMS16/1
  [VR1SEC] -> Scope4/1, RMS18/1  "VR1"
  [VR2SEC] -> Scope4/2, RMS19/1  "VR2"
  RMS20/1 -> Scope1/3  "Vcli"
  RMS18/1 -> Scope1/1  "VR1"
  RMS19/1 -> Scope1/2  "VR2"
  [VCli1] -> Scope4/3, RMS20/1  "Vcli"
  connections:
  Three-Phase Series RLC Load9/LConn3 -- Distributed Parameters Line15/RConn3
  Three-Phase Transformer Inductance Matrix Type (Two Windings)1/RConn2 -- Three-Phase Series RLC Load2/LConn2
  Three-Phase V-I Measurement10/RConn3 -- Three-Phase Fault/LConn3 -- Distributed Parameters Line11/LConn3
  Three-Phase Transformer Inductance Matrix Type (Two Windings)2/RConn1 -- Three-Phase V-I Measurement3/LConn1
  Three-Phase V-I Measurement5/RConn3 -- Subsystem3/LConn3
  Distributed Parameters Line15/LConn3 -- Distributed Parameters Line11/RConn3 -- Three-Phase Series RLC Load8/LConn3
  Three-Phase V-I Measurement5/LConn2 -- Three-Phase V-I Measurement3/RConn2 -- Three-Phase V-I Measurement9/LConn2 -- Three-Phase V-I Measurement7/LConn2
  Distributed Parameters Line10/RConn2 -- Distributed Parameters Line12/LConn2 -- Three-Phase Series RLC Load7/LConn2
  Three-Phase Source/RConn1 -- Three-Phase V-I Measurement2/LConn1
  Subsystem3/RConn3 -- Three-Phase Series RLC Branch4/LConn3
  Three-Phase V-I Measurement6/LConn2 -- Three-Phase Series RLC Branch2/RConn2
  Three-Phase Series RLC Branch3/RConn2 -- Three-Phase Series RLC Load3/LConn2
  Three-Phase Transformer Inductance Matrix Type (Two Windings)1/RConn3 -- Three-Phase Series RLC Load2/LConn3
  Three-Phase V-I Measurement/LConn2 -- Three-Phase V-I Measurement1/LConn2 -- Three-Phase V-I Measurement2/RConn2
  Three-Phase Series RLC Branch/LConn3 -- Three-Phase Series RLC Branch2/LConn3 -- Three-Phase Series RLC Branch4/RConn3
  Distributed Parameters Line7/RConn1 -- Three-Phase Series RLC Branch3/LConn1 -- Three-Phase Series RLC Load5/LConn1
  Subsystem3/RConn2 -- Three-Phase Series RLC Branch4/LConn2
  Three-Phase V-I Measurement5/RConn1 -- Subsystem3/LConn1
  Distributed Parameters Line17/LConn1 -- Three-Phase V-I Measurement11/RConn1
  Three-Phase Transformer Inductance Matrix Type (Two Windings)4/RConn1 -- Three-Phase V-I Measurement4/LConn1
  Three-Phase V-I Measurement8/RConn3 -- Distributed Parameters Line7/LConn3
  Three-Phase Series RLC Load8/LConn2 -- Distributed Parameters Line11/RConn2 -- Distributed Parameters Line15/LConn2
  Three-Phase V-I Measurement9/RConn3 -- Distributed Parameters Line10/LConn3
  Three-Phase V-I Measurement3/RConn1 -- Three-Phase V-I Measurement9/LConn1 -- Three-Phase V-I Measurement7/LConn1 -- Three-Phase V-I Measurement5/LConn1
  Three-Phase Series RLC Branch3/RConn1 -- Three-Phase Series RLC Load3/LConn1
  Load Flow Bus3/LConn1 -- Three-Phase Transformer Inductance Matrix Type (Two Windings)1/RConn1 -- Three-Phase Series RLC Load2/LConn1
  Three-Phase Series RLC Branch3/RConn3 -- Three-Phase Series RLC Load3/LConn3
  Three-Phase Transformer Inductance Matrix Type (Two Windings)4/LConn1 -- Three-Phase V-I Measurement1/RConn1
  Three-Phase V-I Measurement5/RConn2 -- Subsystem3/LConn2
  Three-Phase V-I Measurement5/LConn3 -- Three-Phase V-I Measurement7/LConn3 -- Three-Phase V-I Measurement9/LConn3 -- Three-Phase V-I Measurement3/RConn3
  Subsystem3/RConn1 -- Three-Phase Series RLC Branch4/LConn1
  Three-Phase Transformer Inductance Matrix Type (Two Windings)4/RConn2 -- Three-Phase V-I Measurement4/LConn2
  Three-Phase Series RLC Branch4/RConn1 -- Three-Phase Series RLC Branch/LConn1 -- Three-Phase Series RLC Branch2/LConn1
  Three-Phase Transformer Inductance Matrix Type (Two Windings)4/RConn3 -- Three-Phase V-I Measurement4/LConn3
  Three-Phase V-I Measurement3/LConn3 -- Three-Phase Transformer Inductance Matrix Type (Two Windings)2/RConn3
  Distributed Parameters Line12/RConn3 -- Distributed Parameters Line21/LConn3
  Three-Phase Series RLC Load1/LConn1 -- Three-Phase Series RLC Branch1/LConn1 -- Three-Phase Series RLC Branch/RConn1
  Distributed Parameters Line10/RConn3 -- Distributed Parameters Line12/LConn3 -- Three-Phase Series RLC Load7/LConn3
  Three-Phase V-I Measurement2/RConn1 -- Load Flow Bus/LConn1 -- Three-Phase V-I Measurement/LConn1 -- Three-Phase V-I Measurement1/LConn1
  Three-Phase Source/RConn2 -- Three-Phase V-I Measurement2/LConn2
  Three-Phase Source/RConn3 -- Three-Phase V-I Measurement2/LConn3
  Three-Phase V-I Measurement4/RConn1 -- Three-Phase V-I Measurement11/LConn1 -- Three-Phase V-I Measurement10/LConn1 -- Three-Phase V-I Measurement8/LConn1
  Distributed Parameters Line21/RConn2 -- Three-Phase Series RLC Load6/LConn2
  Three-Phase Transformer Inductance Matrix Type (Two Windings)2/RConn2 -- Three-Phase V-I Measurement3/LConn2
  Three-Phase Transformer Inductance Matrix Type (Two Windings)4/LConn2 -- Three-Phase V-I Measurement1/RConn2
  Three-Phase Series RLC Load9/LConn2 -- Distributed Parameters Line15/RConn2
  Three-Phase Transformer Inductance Matrix Type (Two Windings)4/LConn3 -- Three-Phase V-I Measurement1/RConn3
  Three-Phase Series RLC Branch/LConn2 -- Three-Phase Series RLC Branch4/RConn2 -- Three-Phase Series RLC Branch2/LConn2
  Three-Phase Series RLC Load1/LConn2 -- Three-Phase Series RLC Branch1/LConn2 -- Three-Phase Series RLC Branch/RConn2
  Three-Phase Series RLC Load1/LConn3 -- Three-Phase Series RLC Branch1/LConn3 -- Three-Phase Series RLC Branch/RConn3
  Three-Phase V-I Measurement6/LConn1 -- Three-Phase Series RLC Branch2/RConn1
  Three-Phase Transformer Inductance Matrix Type (Two Windings)1/LConn2 -- Three-Phase V-I Measurement6/RConn2
  Three-Phase Series RLC Load/LConn1 -- Three-Phase Series RLC Branch1/RConn1
  Three-Phase Transformer Inductance Matrix Type (Two Windings)1/LConn1 -- Three-Phase V-I Measurement6/RConn1
  Three-Phase V-I Measurement6/LConn3 -- Three-Phase Series RLC Branch2/RConn3
  Three-Phase Series RLC Load8/LConn1 -- Distributed Parameters Line11/RConn1 -- Distributed Parameters Line15/LConn1
  Three-Phase V-I Measurement7/RConn1 -- Distributed Parameters Line4/LConn1
  Three-Phase V-I Measurement/LConn3 -- Three-Phase V-I Measurement1/LConn3 -- Three-Phase V-I Measurement2/RConn3
  Three-Phase V-I Measurement7/RConn2 -- Distributed Parameters Line4/LConn2
  Distributed Parameters Line7/RConn2 -- Three-Phase Series RLC Branch3/LConn2 -- Three-Phase Series RLC Load5/LConn2
  Three-Phase V-I Measurement8/RConn1 -- Distributed Parameters Line7/LConn1
  Three-Phase Series RLC Load/LConn2 -- Three-Phase Series RLC Branch1/RConn2
  Three-Phase V-I Measurement9/RConn1 -- Distributed Parameters Line10/LConn1
  Distributed Parameters Line17/LConn3 -- Three-Phase V-I Measurement11/RConn3
  Distributed Parameters Line17/RConn3 -- Three-Phase Series RLC Load10/LConn3
  Three-Phase V-I Measurement8/LConn3 -- Three-Phase V-I Measurement10/LConn3 -- Three-Phase V-I Measurement11/LConn3 -- Three-Phase V-I Measurement4/RConn3
  Three-Phase V-I Measurement9/RConn2 -- Distributed Parameters Line10/LConn2
  Distributed Parameters Line17/LConn2 -- Three-Phase V-I Measurement11/RConn2
  Three-Phase V-I Measurement8/RConn2 -- Distributed Parameters Line7/LConn2
  Three-Phase V-I Measurement10/RConn1 -- Three-Phase Fault/LConn1 -- Distributed Parameters Line11/LConn1
  Distributed Parameters Line11/LConn2 -- Three-Phase Fault/LConn2 -- Three-Phase V-I Measurement10/RConn2
  Distributed Parameters Line12/LConn1 -- Distributed Parameters Line10/RConn1 -- Three-Phase Series RLC Load7/LConn1
  Distributed Parameters Line12/RConn1 -- Distributed Parameters Line21/LConn1
  Distributed Parameters Line12/RConn2 -- Distributed Parameters Line21/LConn2
  Distributed Parameters Line21/RConn3 -- Three-Phase Series RLC Load6/LConn3
  Three-Phase Series RLC Load5/LConn3 -- Distributed Parameters Line7/RConn3 -- Three-Phase Series RLC Branch3/LConn3
  Three-Phase Transformer Inductance Matrix Type (Two Windings)2/LConn3 -- Three-Phase V-I Measurement/RConn3
  Three-Phase Transformer Inductance Matrix Type (Two Windings)2/LConn2 -- Three-Phase V-I Measurement/RConn2
  Three-Phase V-I Measurement8/LConn2 -- Three-Phase V-I Measurement10/LConn2 -- Three-Phase V-I Measurement11/LConn2 -- Three-Phase V-I Measurement4/RConn2
  Three-Phase Series RLC Load/LConn3 -- Three-Phase Series RLC Branch1/RConn3
  Distributed Parameters Line17/RConn1 -- Three-Phase Series RLC Load10/LConn1
  Three-Phase Series RLC Load9/LConn1 -- Distributed Parameters Line15/RConn1
  Three-Phase Series RLC Load4/LConn3 -- Distributed Parameters Line4/RConn3
  Three-Phase Series RLC Load4/LConn2 -- Distributed Parameters Line4/RConn2
  Three-Phase Transformer Inductance Matrix Type (Two Windings)2/LConn1 -- Three-Phase V-I Measurement/RConn1
  Three-Phase V-I Measurement7/RConn3 -- Distributed Parameters Line4/LConn3
  Three-Phase Series RLC Load10/LConn2 -- Distributed Parameters Line17/RConn2
  Three-Phase Transformer Inductance Matrix Type (Two Windings)1/LConn3 -- Three-Phase V-I Measurement6/RConn3
  Three-Phase Series RLC Load4/LConn1 -- Distributed Parameters Line4/RConn1
  Distributed Parameters Line21/RConn1 -- Three-Phase Series RLC Load6/LConn1
